simulink model "article_implementation"  (R2020b)
settings: Solver=VariableStepAuto  StartTime=0.0  StopTime=30  RelTol=1e-3
values from neighbouring files (symbols this model uses):
  C = [1 0 0 ;0 1 0 ]    [experinces.m]    (also in main.m = [eye(3), zeros(3,3)])
  Q = diag([0 0.005 1*10^-4 ])    [experinces.m]    (also in main.m = [Q_w, zeros(3,3);zeros(3,3), Q_b])
  R = diag([0.0005/150 0.05/150])    [experinces.m]    (also in main.m = eye(3)*0.005)
settings Model: Creator=renato  LastModifiedBy=renato

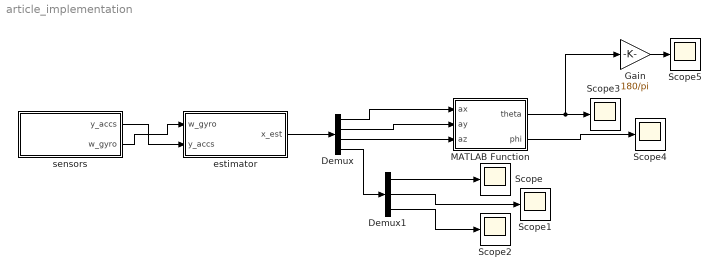
== system article_implementation ==
  Demux : Demux  Outputs=[1 1 1 3]
  Demux1 : Demux  Outputs=[1 1 1]
  Gain : Gain  Gain=180/pi
  MATLAB Function : MATLAB Function  TreatAsAtomicUnit=on
  Scope{,1..5} (6 alike) : Scope
  estimator : Subsystem
  sensors : Subsystem
  wires:
  estimator/1(x_est) -> Demux/1
  Demux/1 -> MATLAB Function/1(ax)
  Demux/2 -> MATLAB Function/2(ay)
  Demux/3 -> MATLAB Function/3(az)
  Demux/4 -> Demux1/1
  Demux1/1 -> Scope/1
  Demux1/2 -> Scope1/1
  Demux1/3 -> Scope2/1
  MATLAB Function/1(theta) -> Gain/1, Scope3/1
  MATLAB Function/2(phi) -> Scope4/1
  sensors/1(y_accs) -> estimator/2(y_accs)
  sensors/2(w_gyro) -> estimator/1(w_gyro)
  Gain/1 -> Scope5/1

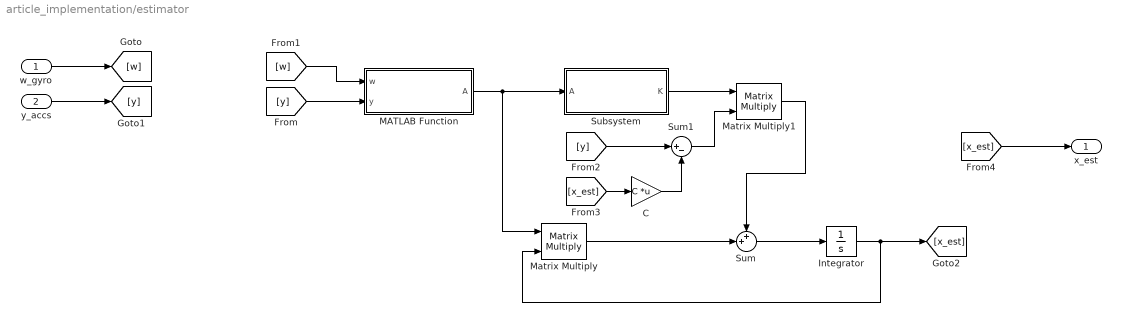
== system article_implementation/estimator ==
  w_gyro : Inport
  y_accs : Inport  Port=2
  C : Gain  Gain=C  Multiplication=Matrix(K*u)
  Integrator : Integrator
  MATLAB Function : MATLAB Function  TreatAsAtomicUnit=on
  Matrix Multiply : Product  Multiplication=Matrix(*)
  Matrix Multiply1 : Product  Multiplication=Matrix(*)
  Subsystem : Subsystem
  Sum : Sum  Inputs=++|
  Sum1 : Sum  Inputs=|+-
  x_est : Outport
  wires:
  Integrator/1 -> [x_est], Matrix Multiply/2
  Subsystem/1(K) -> Matrix Multiply1/1
  [x_est] -> C/1
  C/1 -> Sum1/2
  Sum/1 -> Integrator/1
  [y] -> MATLAB Function/2(y)
  [w] -> MATLAB Function/1(w)
  [y] -> Sum1/1
  Matrix Multiply1/1 -> Sum/1
  Sum1/1 -> Matrix Multiply1/2
  Matrix Multiply/1 -> Sum/2
  MATLAB Function/1(A) -> Subsystem/1(A), Matrix Multiply/1
  [x_est] -> x_est/1
  w_gyro/1 -> [w]
  y_accs/1 -> [y]

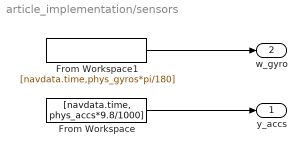
== system article_implementation/sensors ==
  From Workspace : FromWorkspace  VariableName=[navdata.time, phys_accs*9.8/1000]
  From Workspace1 : FromWorkspace  VariableName=[navdata.time,phys_gyros*pi/180]
  y_accs : Outport
  w_gyro : Outport  Port=2
  wires:
  From Workspace1/1 -> w_gyro/1
  From Workspace/1 -> y_accs/1

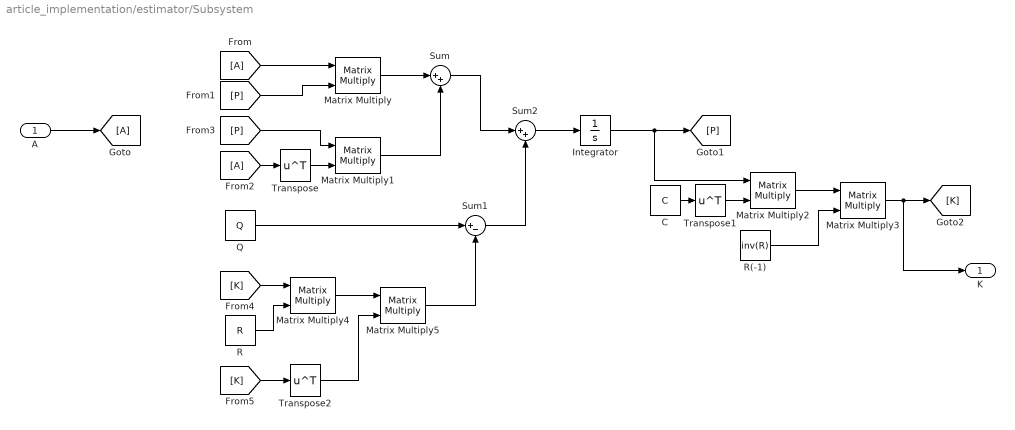
== system article_implementation/estimator/Subsystem ==
  A : Inport
  C : Constant  Value=C
  Integrator : Integrator  InitialCondition=eye(6)
  Matrix Multiply{,1..5} (6 alike) : Product  Multiplication=Matrix(*)
  Q : Constant  Value=Q
  R : Constant  Value=R
  R(-1) : Constant  Value=inv(R)
  Sum : Sum  Inputs=|++
  Sum1 : Sum  Inputs=|+-
  Sum2 : Sum  Inputs=|++
  Transpose : Math  Operator=transpose  SaturateOnIntegerOverflow=on
  Transpose1 : Math  Operator=transpose  SaturateOnIntegerOverflow=on
  Transpose2 : Math  Operator=transpose  SaturateOnIntegerOverflow=on
  K : Outport
  wires:
  A/1 -> [A]
  Integrator/1 -> Matrix Multiply2/1, [P]
  [A] -> Matrix Multiply/1
  [P] -> Matrix Multiply/2
  [A] -> Transpose/1
  Transpose/1 -> Matrix Multiply1/2
  [P] -> Matrix Multiply1/1
  Transpose1/1 -> Matrix Multiply2/2
  C/1 -> Transpose1/1
  Matrix Multiply2/1 -> Matrix Multiply3/1
  R(-1)/1 -> Matrix Multiply3/2
  Matrix Multiply3/1 -> K/1, [K]
  [K] -> Transpose2/1
  [K] -> Matrix Multiply4/1
  R/1 -> Matrix Multiply4/2
  Matrix Multiply4/1 -> Matrix Multiply5/1
  Transpose2/1 -> Matrix Multiply5/2
  Matrix Multiply/1 -> Sum/1
  Matrix Multiply1/1 -> Sum/2
  Q/1 -> Sum1/1
  Matrix Multiply5/1 -> Sum1/2
  Sum/1 -> Sum2/1
  Sum1/1 -> Sum2/2
  Sum2/1 -> Integrator/1

== matlab function article_implementation/MATLAB Function ==
  data: ax input; theta output; ay input; az input; phi output
function [theta, phi] = fcn(ax,ay,az)
    % need to see if the formulas are right
    theta=atan2(ax, sqrt(az^2 + ay^2));
    phi=atan2(ay,az);

end

== matlab function article_implementation/estimator/MATLAB Function ==
  data: w input; A output; y input
function A = calculate_A(w, y)
    aux1 = -[0, -w(3), w(2); 
             w(3), 0, -w(1);
             -w(2), w(1), 0];
    aux2 = [0, -y(3), y(2);
            y(3), 0, -y(1);
            -y(2), y(1), 0];   
    
A = [aux1 , aux2; zeros(3), zeros(3)];
